simulink model "WEC_Sim_Driver"  (R2013a)
settings: Solver=ode4  StartTime=StartTime  StopTime=EndTime  FixedStep=deltaT  MaxStep=deltaTMax  MinStep=deltaTMin  RelTol=1e-3
undefined symbols (not defined in the file): A_bore, A_c_F, A_c_P, A_rod, angle_arm_aft, Bd, C_aft, deltaT, Gen_Damp, hyd_mot_eff, hydro, hydroForce, Jtot, K_aft, Kd, mooring_c, mooring_k, nonlinear_params, omega_s, p_atm, p_hp, p_lp, pump_vol_eff, r_g, STLfloat, STLplate, Ts, V_hp, V_lp, Vg, X, Y, Z
libraries: nesl_utility x35, sm_lib x14
(part 2 of 2)

== matlab function WEC_Sim_Driver/Structure2/Convert ==
  data: Q input; E output
function E  = EulerAngle(Q)
%#codegen
E=zeros(3,1);
E(1) = atan( (2*(Q(1)*Q(2)+Q(3)*Q(4))) / (1-2* (Q(2)^2+Q(3)^2) ) );
E(2) = asin( 2* (Q(1)*Q(3) - Q(4)*Q(2)));
E(3) = atan( (2*(Q(1)*Q(4)+Q(2)*Q(3))) / (1-2* (Q(3)^2+Q(4)^2) ) );

== matlab function WEC_Sim_Driver/Structure2/Convert1 ==
  data: Q input; E output
function E  = EulerAngle(Q)
%#codegen
E=zeros(3,1);
E(1) = atan( (2*(Q(1)*Q(2)+Q(3)*Q(4))) / (1-2* (Q(2)^2+Q(3)^2) ) );
E(2) = asin( 2* (Q(1)*Q(3) - Q(4)*Q(2)));
E(3) = atan( (2*(Q(1)*Q(4)+Q(2)*Q(3))) / (1-2* (Q(3)^2+Q(4)^2) ) );

== matlab function WEC_Sim_Driver/Structure2/Convert2 ==
  data: Q input; E output
function E  = EulerAngle(Q)
%#codegen
E=zeros(3,1);
E(1) = atan( (2*(Q(1)*Q(2)+Q(3)*Q(4))) / (1-2* (Q(2)^2+Q(3)^2) ) );
E(2) = asin( 2* (Q(1)*Q(3) - Q(4)*Q(2)));
E(3) = atan( (2*(Q(1)*Q(4)+Q(2)*Q(3))) / (1-2* (Q(3)^2+Q(4)^2) ) );

== matlab function WEC_Sim_Driver/Linear HydroForce2/MATLAB Function ==
  data: t input; F output; deltaT input; matrix input
function F  = ExcitationLookup(t,deltaT,matrix)

int=round(t/deltaT+1);
F=matrix(int,:)';

== matlab function WEC_Sim_Driver/Fully-Nonlinear HydroForce2/Linear Excitation ==
  data: t input; F output; deltaT input; matrix input
function F  = ExcitationLookup(t,deltaT,matrix)

int=round(t/deltaT+1);
F=matrix(int,:)';

== matlab function WEC_Sim_Driver/Fully-Nonlinear HydroForce1/Fully-Nonlinear Hydrostatic Restoring and Excitation/Body1 Nonlinear Restoring and Excitation ==
  data: STL input; t input; BodyForce output; Disp input; BodyMoment output; nonlinear_params input; psi_m output; p_FK_total output; p_FK_l_total output
function [BodyForce,BodyMoment,psi_m,p_FK_total,p_FK_l_total] = vectorbuoyancy(STL, t,Disp,nonlinear_params)
%STL(a,b,c)  where a denotes the triangle, b denotes the point (1-3) and c
%            denotes the component (x, y or z)
%dZ          a scalar value describing HEAVE
%axisRot     a vector describing the axis about which the body is rotated
%angleRot    the angle by which the body is rotated about axisRot
%refZ        the location of the

% algorithm for point rotation from http://paulbourke.net/geometry/rotate/
% algorithm for volume calc from
% http://stackoverflow.com/questions/1406029/how-to-calculate-the-volume-of-a-3d-mesh-object-the-surface-of-which-is-made-up
% via  http://amp.ece.cmu.edu/Publication/Cha/icip01_Cha.pdf

%determine size of STL
[a b c] = size(STL);

%make sure angleRot is a unit vector
% magAR = sqrt(axisRot(1)^2 + axisRot(2)^2 + axisRot(3)^2);
% axisRot = axisRot/magAR;
axisRotx=[1 0 0];
axisRoty=[0 1 0];
dX=Disp(1);
dZ=Disp(3);
angleRotx=Disp(4);
angleRoty=Disp(5);
Amp=nonlinear_params(1);
k=nonlinear_params(2);
w=nonlinear_params(3);
d=nonlinear_params(4);
psi = zeros(a,b);
psi_l= zeros(a,b);
psi_m = 0;
psi_avg = zeros(a,b);
psi_l_avg = zeros(a,b);
STL_l=zeros(size(STL));

% Fix body at mean water level for linear buoyancy & excitation calc
for i=1:1:a
    for j=1:1:3
        q_l = zeros(1,3);
            %plunge object
            q_l(1) = STL(i,j,1);
            q_l(2) = STL(i,j,2);
            q_l(3) = STL(i,j,3) -17.606;
        if q_l(3) > 0
            q_l(3) = 0;
        end
        psi_l(i,j) =Amp*cos(k*(q_l(1)+dX)-w*t);
        %save altered point
        STL_l(i,j,:) = q_l;
    end
end

% Rotate and translate body for nonlinear buoyancy & excitation calc
for i=1:1:a
    for j=1:1:3
        q = zeros(1,3);
        
        %Calculate water height near body CG before moving body
        if STL(i,j,1)<0.001
            psi_m=Amp*cos(k*(dX)-w*t);
        end
        
%         perform y-direction rotation
        if angleRoty ~= 0
            
            costhetay = cos(angleRoty);
            sinthetay = sin(angleRoty);
            
            q(1) = q(1) + (costhetay + (1 - costhetay) * axisRoty(1) * axisRoty(1)) * STL(i,j,1);
            q(1) = q(1) + ((1 - costhetay) * axisRoty(1) * axisRoty(2) - axisRoty(3) * sinthetay) * STL(i,j,2);
            q(1) = q(1) + ((1 - costhetay) * axisRoty(1) * axisRoty(3) + axisRoty(2) * sinthetay) * STL(i,j,3);
            
            q(2) = q(2) + ((1 - costhetay) * axisRoty(1) * axisRoty(2) + axisRoty(3) * sinthetay) * STL(i,j,1);
            q(2) = q(2) + (costhetay + (1 - costhetay) * axisRoty(2) * axisRoty(2)) * STL(i,j,2);
            q(2) = q(2) + ((1 - costhetay) * axisRoty(2) * axisRoty(3) - axisRoty(1) * sinthetay) * STL(i,j,3);
            
            q(3) = q(3) + ((1 - costhetay) * axisRoty(1) * axisRoty(3) - axisRoty(2) * sinthetay) * STL(i,j,1);
            q(3) = q(3) + ((1 - costhetay) * axisRoty(2) * axisRoty(3) + axisRoty(1) * sinthetay) * STL(i,j,2);
            q(3) = q(3) + (costhetay + (1 - costhetay) * axisRoty(3) * axisRoty(3)) * STL(i,j,3);
            
%             q(3) = q(3) + dZ(1);
        end
        if angleRoty ~= 0
        %save altered point
        STL(i,j,:) = q;
        end
    end
end

for i=1:1:a
    for j=1:1:3
        q = zeros(1,3);
%         %perform x-direction rotation
        if angleRotx ~= 0
            
            costhetax = cos(angleRotx);
            sinthetax = sin(angleRotx);
            
            q(1) = q(1) + (costhetax + (1 - costhetax) * axisRotx(1) * axisRotx(1)) * STL(i,j,1);
            q(1) = q(1) + ((1 - costhetax) * axisRotx(1) * axisRotx(2) - axisRotx(3) * sinthetax) * STL(i,j,2);
            q(1) = q(1) + ((1 - costhetax) * axisRotx(1) * axisRotx(3) + axisRotx(2) * sinthetax) * STL(i,j,3);
            
            q(2) = q(2) + ((1 - costhetax) * axisRotx(1) * axisRotx(2) + axisRotx(3) * sinthetax) * STL(i,j,1);
            q(2) = q(2) + (costhetax + (1 - costhetax) * axisRotx(2) * axisRotx(2)) * STL(i,j,2);
            q(2) = q(2) + ((1 - costhetax) * axisRotx(2) * axisRotx(3) - axisRotx(1) * sinthetax) * STL(i,j,3);
            
            q(3) = q(3) + ((1 - costhetax) * axisRotx(1) * axisRotx(3) - axisRotx(2) * sinthetax) * STL(i,j,1);
            q(3) = q(3) + ((1 - costhetax) * axisRotx(2) * axisRotx(3) + axisRotx(1) * sinthetax) * STL(i,j,2);
            q(3) = q(3) + (costhetax + (1 - costhetax) * axisRotx(3) * axisRotx(3)) * STL(i,j,3);
            
            q(3) = q(3) + dZ(1);
        else
            %plunge object
            q(1) = STL(i,j,1);
            q(2) = STL(i,j,2);
            q(3) = STL(i,j,3) + dZ(1);
        end
        
        %Truncate at instantaneous free surface
        psi(i,j) =Amp*cos(k*(q(1)+ dX)-w*t);
        if q(3) > psi(i,j)
            q(3) = psi(i,j);
        end
        
        %Truncate at instantaneous free surface
%         if q(3) > 0
%             q(3) = 0;
%         end
        
        %save altered point
        STL(i,j,:) = q;
    end
end

%Calculate buoyancy force and restoring moments
BodyForce=zeros(3,1);
BodyMoment=zeros(3,1);
p_FK_total=zeros(3,1);
p_FK_l_total=zeros(3,1);
for i=1:1:a
    x_m=(STL(i,1,1)+STL(i,2,1)+STL(i,3,1))/3;        %z coordinate for panel center
    y_m=(STL(i,1,2)+STL(i,2,2)+STL(i,3,2))/3;        %z coordinate for panel center
    z_m=(STL(i,1,3)+STL(i,2,3)+STL(i,3,3))/3;        %z coordinate for panel center
    r_m=[x_m; y_m; z_m];
        
    r_a=[STL(i,1,1); STL(i,1,2); STL(i,1,3)];             %vector describing location of panel's A vertex
    r_b=[STL(i,2,1); STL(i,2,2); STL(i,2,3)];             %vector describing location of panel's B vertex
    r_c=[STL(i,3,1); STL(i,3,2); STL(i,3,3)];             %vector describing location of panel's C vertex
 
    AB=r_b-r_a;
    AC=r_c-r_a;
    CP=cross(AC,AB);
    area=.5*CP;
    
    x_m_l=(STL_l(i,1,1)+STL_l(i,2,1)+STL_l(i,3,1))/3;        %z coordinate for panel center
    y_m_l=(STL_l(i,1,2)+STL_l(i,2,2)+STL_l(i,3,2))/3;        %z coordinate for panel center
    z_m_l=(STL_l(i,1,3)+STL_l(i,2,3)+STL_l(i,3,3))/3;        %z coordinate for panel center
    r_m_l=[x_m_l; y_m_l; z_m_l];  
    
    r_a_l=[STL_l(i,1,1); STL_l(i,1,2); STL_l(i,1,3)];             %vector describing location of panel's A vertex
    r_b_l=[STL_l(i,2,1); STL_l(i,2,2); STL_l(i,2,3)];             %vector describing location of panel's B vertex
    r_c_l=[STL_l(i,3,1); STL_l(i,3,2); STL_l(i,3,3)];             %vector describing location of panel's C verte
      
    AB_l=r_b_l-r_a_l;
    AC_l=r_c_l-r_a_l;
    CP_l=cross(AC_l,AB_l);
    area_l=.5*CP_l;
    
    psi_avg = (psi(i,1)+psi(i,2)+psi(i,3))/3;
    psi_l_avg = (psi_l(i,1)+psi_l(i,2)+psi_l(i,3))/3;
    
    p_HS=-z_m*area;
    p_FK=area*psi_avg*cosh(k*(z_m+psi_avg+d))/cosh(k*d);
    p_FK_l=area_l*psi_l_avg*cosh(k*(z_m_l+psi_l_avg+d))/cosh(k*d);
    p_total=p_HS+p_FK-p_FK_l;
    
    BodyForce=BodyForce+p_total;
    PanelMoment=cross(r_m,p_total);
    BodyMoment=BodyMoment+PanelMoment;

    p_FK_total=p_FK_total+p_FK;
    p_FK_l_total=p_FK_l_total+p_FK_l;
end
% BodyForce(1)=0;
% BodyForce(2)=0;
% BodyMoment(1)=-0.05*angleRot(1);
% BodyMoment(3)=-50000*angleRot(3);

== matlab function WEC_Sim_Driver/Fully-Nonlinear HydroForce1/Linear Excitation ==
  data: t input; F output; deltaT input; matrix input
function F  = ExcitationLookup(t,deltaT,matrix)

int=round(t/deltaT+1);
F=matrix(int,:)';

== matlab function WEC_Sim_Driver/Quasi-Nonlinear HydroForce2/Linear Excitation ==
  data: t input; F output; deltaT input; matrix input
function F  = ExcitationLookup(t,deltaT,matrix)

int=round(t/deltaT+1);
F=matrix(int,:)';

== matlab function WEC_Sim_Driver/Quasi-Nonlinear HydroForce2/Quasi-Nonlinear Hydrostatic Restoring/Submerged Volume ==
  data: STL input; BodyForce output; Disp2 input; BodyMoment output; TotalArea output; PanelForce output
function [BodyForce,BodyMoment,TotalArea,PanelForce] = vectorbuoyancy(STL, Disp2)
%STL(a,b,c)  where a denotes the triangle, b denotes the point (1-3) and c
%            denotes the component (x, y or z)
%dZ          a scalar value describing HEAVE
%axisRot     a vector describing the axis about which the body is rotated
%angleRot    the angle by which the body is rotated about axisRot
%refZ        the location of the

% algorithm for point rotation from http://paulbourke.net/geometry/rotate/
% algorithm for volume calc from
% http://stackoverflow.com/questions/1406029/how-to-calculate-the-volume-of-a-3d-mesh-object-the-surface-of-which-is-made-up
% via  http://amp.ece.cmu.edu/Publication/Cha/icip01_Cha.pdf

%determine size of STL
[a b c] = size(STL);

%make sure angleRot is a unit vector
% magAR = sqrt(axisRot(1)^2 + axisRot(2)^2 + axisRot(3)^2);
% axisRot = axisRot/magAR;
axisRotx=[1 0 0];
axisRoty=[0 1 0];
dZ=Disp2(3);
angleRotx=Disp2(4);
angleRoty=Disp2(5);

% update locations of points
for i=1:1:a
    for j=1:1:3
        q = zeros(1,3);
        
%         perform y-direction rotation
        if angleRoty ~= 0
            
            costhetay = cos(angleRoty);
            sinthetay = sin(angleRoty);
            
            q(1) = q(1) + (costhetay + (1 - costhetay) * axisRoty(1) * axisRoty(1)) * STL(i,j,1);
            q(1) = q(1) + ((1 - costhetay) * axisRoty(1) * axisRoty(2) - axisRoty(3) * sinthetay) * STL(i,j,2);
            q(1) = q(1) + ((1 - costhetay) * axisRoty(1) * axisRoty(3) + axisRoty(2) * sinthetay) * STL(i,j,3);
            
            q(2) = q(2) + ((1 - costhetay) * axisRoty(1) * axisRoty(2) + axisRoty(3) * sinthetay) * STL(i,j,1);
            q(2) = q(2) + (costhetay + (1 - costhetay) * axisRoty(2) * axisRoty(2)) * STL(i,j,2);
            q(2) = q(2) + ((1 - costhetay) * axisRoty(2) * axisRoty(3) - axisRoty(1) * sinthetay) * STL(i,j,3);
            
            q(3) = q(3) + ((1 - costhetay) * axisRoty(1) * axisRoty(3) - axisRoty(2) * sinthetay) * STL(i,j,1);
            q(3) = q(3) + ((1 - costhetay) * axisRoty(2) * axisRoty(3) + axisRoty(1) * sinthetay) * STL(i,j,2);
            q(3) = q(3) + (costhetay + (1 - costhetay) * axisRoty(3) * axisRoty(3)) * STL(i,j,3);
            
%             q(3) = q(3) + dZ(1);
        end
        if angleRoty ~= 0
        %save altered point
        STL(i,j,:) = q;
        end
    end
end

for i=1:1:a
    for j=1:1:3
        q = zeros(1,3);
%         %perform x-direction rotation
        if angleRotx ~= 0
            
            costhetax = cos(angleRotx);
            sinthetax = sin(angleRotx);
            
            q(1) = q(1) + (costhetax + (1 - costhetax) * axisRotx(1) * axisRotx(1)) * STL(i,j,1);
            q(1) = q(1) + ((1 - costhetax) * axisRotx(1) * axisRotx(2) - axisRotx(3) * sinthetax) * STL(i,j,2);
            q(1) = q(1) + ((1 - costhetax) * axisRotx(1) * axisRotx(3) + axisRotx(2) * sinthetax) * STL(i,j,3);
            
            q(2) = q(2) + ((1 - costhetax) * axisRotx(1) * axisRotx(2) + axisRotx(3) * sinthetax) * STL(i,j,1);
            q(2) = q(2) + (costhetax + (1 - costhetax) * axisRotx(2) * axisRotx(2)) * STL(i,j,2);
            q(2) = q(2) + ((1 - costhetax) * axisRotx(2) * axisRotx(3) - axisRotx(1) * sinthetax) * STL(i,j,3);
            
            q(3) = q(3) + ((1 - costhetax) * axisRotx(1) * axisRotx(3) - axisRotx(2) * sinthetax) * STL(i,j,1);
            q(3) = q(3) + ((1 - costhetax) * axisRotx(2) * axisRotx(3) + axisRotx(1) * sinthetax) * STL(i,j,2);
            q(3) = q(3) + (costhetax + (1 - costhetax) * axisRotx(3) * axisRotx(3)) * STL(i,j,3);
            
            q(3) = q(3) + dZ(1);
        else
            %plunge object
            q(1) = STL(i,j,1);
            q(2) = STL(i,j,2);
            q(3) = STL(i,j,3) + dZ(1);
        end
        
        %truncate at water surface
        if q(3) > 0
            q(3) = 0;
        end
        
        %save altered point
        STL(i,j,:) = q;
    end
end

%Calculate buoyancy force and restoring moments
BodyForce=zeros(3,1);
BodyMoment=zeros(3,1);
TotalArea=zeros(3,1);
for i=1:1:a
    x_m=(STL(i,1,1)+STL(i,2,1)+STL(i,3,1))/3;        %z coordinate for panel center
    y_m=(STL(i,1,2)+STL(i,2,2)+STL(i,3,2))/3;        %z coordinate for panel center
    z_m=(STL(i,1,3)+STL(i,2,3)+STL(i,3,3))/3;        %z coordinate for panel center
    r_m=[x_m; y_m; z_m];
        
    r_a=[STL(i,1,1); STL(i,1,2); STL(i,1,3)];             %vector describing location of panel's A vertex
    r_b=[STL(i,2,1); STL(i,2,2); STL(i,2,3)];             %vector describing location of panel's B vertex
    r_c=[STL(i,3,1); STL(i,3,2); STL(i,3,3)];             %vector describing location of panel's C vertex
 
    AB=r_b-r_a;
    AC=r_c-r_a;
    CP=cross(AC,AB);
    area=.5*CP;
    
    PanelForce=-z_m*area;
    BodyForce=BodyForce+PanelForce;
    
    PanelMoment=cross(r_m,PanelForce);
    BodyMoment=BodyMoment+PanelMoment;
    TotalArea=TotalArea+area;
end

% BodyForce(1)=0;
% BodyForce(2)=0;
% BodyMoment(1)=-0.05*angleRot(1);
% BodyMoment(3)=-50000*angleRot(3);

== matlab function WEC_Sim_Driver/Fully-Nonlinear HydroForce2/Fully-Nonlinear Hydrostatic Restoring and Excitation/Body1 Nonlinear Restoring and Excitation ==
  data: STL input; t input; BodyForce output; Disp2 input; BodyMoment output; nonlinear_params input; psi_m output; p_FK_total output; p_FK_l_total output
function [BodyForce,BodyMoment,psi_m,p_FK_total,p_FK_l_total] = vectorbuoyancy(STL, t,Disp2,nonlinear_params)
%STL(a,b,c)  where a denotes the triangle, b denotes the point (1-3) and c
%            denotes the component (x, y or z)
%dZ          a scalar value describing HEAVE
%axisRot     a vector describing the axis about which the body is rotated
%angleRot    the angle by which the body is rotated about axisRot
%refZ        the location of the

% algorithm for point rotation from http://paulbourke.net/geometry/rotate/
% algorithm for volume calc from
% http://stackoverflow.com/questions/1406029/how-to-calculate-the-volume-of-a-3d-mesh-object-the-surface-of-which-is-made-up
% via  http://amp.ece.cmu.edu/Publication/Cha/icip01_Cha.pdf

%determine size of STL
[a b c] = size(STL);

%make sure angleRot is a unit vector
% magAR = sqrt(axisRot(1)^2 + axisRot(2)^2 + axisRot(3)^2);
% axisRot = axisRot/magAR;
axisRotx=[1 0 0];
axisRoty=[0 1 0];
dX=Disp2(1);
dZ=Disp2(3);
angleRotx=Disp2(4);
angleRoty=Disp2(5);
Amp=nonlinear_params(1);
k=nonlinear_params(2);
w=nonlinear_params(3);
d=nonlinear_params(4);
psi = zeros(a,b);
psi_l= zeros(a,b);
psi_m = 0;
psi_avg = zeros(a,b);
psi_l_avg = zeros(a,b);
STL_l=zeros(size(STL));

% Fix body at mean water level for linear buoyancy & excitation calc
for i=1:1:a
    for j=1:1:3
        q_l = zeros(1,3);
            %plunge object
            q_l(1) = STL(i,j,1);
            q_l(2) = STL(i,j,2);
            q_l(3) = STL(i,j,3) -17.606;
        if q_l(3) > 0
            q_l(3) = 0;
        end
        psi_l(i,j) =Amp*cos(k*(q_l(1)+dX)-w*t);
        %save altered point
        STL_l(i,j,:) = q_l;
    end
end

% Rotate and translate body for nonlinear buoyancy & excitation calc
for i=1:1:a
    for j=1:1:3
        q = zeros(1,3);
        
        %Calculate water height near body CG before moving body
        if STL(i,j,1)<0.001
            psi_m=Amp*cos(k*(dX)-w*t);
        end
        
%         perform y-direction rotation
        if angleRoty ~= 0
            
            costhetay = cos(angleRoty);
            sinthetay = sin(angleRoty);
            
            q(1) = q(1) + (costhetay + (1 - costhetay) * axisRoty(1) * axisRoty(1)) * STL(i,j,1);
            q(1) = q(1) + ((1 - costhetay) * axisRoty(1) * axisRoty(2) - axisRoty(3) * sinthetay) * STL(i,j,2);
            q(1) = q(1) + ((1 - costhetay) * axisRoty(1) * axisRoty(3) + axisRoty(2) * sinthetay) * STL(i,j,3);
            
            q(2) = q(2) + ((1 - costhetay) * axisRoty(1) * axisRoty(2) + axisRoty(3) * sinthetay) * STL(i,j,1);
            q(2) = q(2) + (costhetay + (1 - costhetay) * axisRoty(2) * axisRoty(2)) * STL(i,j,2);
            q(2) = q(2) + ((1 - costhetay) * axisRoty(2) * axisRoty(3) - axisRoty(1) * sinthetay) * STL(i,j,3);
            
            q(3) = q(3) + ((1 - costhetay) * axisRoty(1) * axisRoty(3) - axisRoty(2) * sinthetay) * STL(i,j,1);
            q(3) = q(3) + ((1 - costhetay) * axisRoty(2) * axisRoty(3) + axisRoty(1) * sinthetay) * STL(i,j,2);
            q(3) = q(3) + (costhetay + (1 - costhetay) * axisRoty(3) * axisRoty(3)) * STL(i,j,3);
            
%             q(3) = q(3) + dZ(1);
        end
        if angleRoty ~= 0
        %save altered point
        STL(i,j,:) = q;
        end
    end
end

for i=1:1:a
    for j=1:1:3
        q = zeros(1,3);
%         %perform x-direction rotation
        if angleRotx ~= 0
            
            costhetax = cos(angleRotx);
            sinthetax = sin(angleRotx);
            
            q(1) = q(1) + (costhetax + (1 - costhetax) * axisRotx(1) * axisRotx(1)) * STL(i,j,1);
            q(1) = q(1) + ((1 - costhetax) * axisRotx(1) * axisRotx(2) - axisRotx(3) * sinthetax) * STL(i,j,2);
            q(1) = q(1) + ((1 - costhetax) * axisRotx(1) * axisRotx(3) + axisRotx(2) * sinthetax) * STL(i,j,3);
            
            q(2) = q(2) + ((1 - costhetax) * axisRotx(1) * axisRotx(2) + axisRotx(3) * sinthetax) * STL(i,j,1);
            q(2) = q(2) + (costhetax + (1 - costhetax) * axisRotx(2) * axisRotx(2)) * STL(i,j,2);
            q(2) = q(2) + ((1 - costhetax) * axisRotx(2) * axisRotx(3) - axisRotx(1) * sinthetax) * STL(i,j,3);
            
            q(3) = q(3) + ((1 - costhetax) * axisRotx(1) * axisRotx(3) - axisRotx(2) * sinthetax) * STL(i,j,1);
            q(3) = q(3) + ((1 - costhetax) * axisRotx(2) * axisRotx(3) + axisRotx(1) * sinthetax) * STL(i,j,2);
            q(3) = q(3) + (costhetax + (1 - costhetax) * axisRotx(3) * axisRotx(3)) * STL(i,j,3);
            
            q(3) = q(3) + dZ(1);
        else
            %plunge object
            q(1) = STL(i,j,1);
            q(2) = STL(i,j,2);
            q(3) = STL(i,j,3) + dZ(1);
        end
        
        %Truncate at instantaneous free surface
        psi(i,j) =Amp*cos(k*(q(1)+ dX)-w*t);
        if q(3) > psi(i,j)
            q(3) = psi(i,j);
        end
        
        %Truncate at instantaneous free surface
%         if q(3) > 0
%             q(3) = 0;
%         end
        
        %save altered point
        STL(i,j,:) = q;
    end
end

%Calculate buoyancy force and restoring moments
BodyForce=zeros(3,1);
BodyMoment=zeros(3,1);
p_FK_total=zeros(3,1);
p_FK_l_total=zeros(3,1);
for i=1:1:a
    x_m=(STL(i,1,1)+STL(i,2,1)+STL(i,3,1))/3;        %z coordinate for panel center
    y_m=(STL(i,1,2)+STL(i,2,2)+STL(i,3,2))/3;        %z coordinate for panel center
    z_m=(STL(i,1,3)+STL(i,2,3)+STL(i,3,3))/3;        %z coordinate for panel center
    r_m=[x_m; y_m; z_m];
        
    r_a=[STL(i,1,1); STL(i,1,2); STL(i,1,3)];             %vector describing location of panel's A vertex
    r_b=[STL(i,2,1); STL(i,2,2); STL(i,2,3)];             %vector describing location of panel's B vertex
    r_c=[STL(i,3,1); STL(i,3,2); STL(i,3,3)];             %vector describing location of panel's C vertex
 
    AB=r_b-r_a;
    AC=r_c-r_a;
    CP=cross(AC,AB);
    area=.5*CP;
    
    x_m_l=(STL_l(i,1,1)+STL_l(i,2,1)+STL_l(i,3,1))/3;        %z coordinate for panel center
    y_m_l=(STL_l(i,1,2)+STL_l(i,2,2)+STL_l(i,3,2))/3;        %z coordinate for panel center
    z_m_l=(STL_l(i,1,3)+STL_l(i,2,3)+STL_l(i,3,3))/3;        %z coordinate for panel center
    r_m_l=[x_m_l; y_m_l; z_m_l];  
    
    r_a_l=[STL_l(i,1,1); STL_l(i,1,2); STL_l(i,1,3)];             %vector describing location of panel's A vertex
    r_b_l=[STL_l(i,2,1); STL_l(i,2,2); STL_l(i,2,3)];             %vector describing location of panel's B vertex
    r_c_l=[STL_l(i,3,1); STL_l(i,3,2); STL_l(i,3,3)];             %vector describing location of panel's C verte
      
    AB_l=r_b_l-r_a_l;
    AC_l=r_c_l-r_a_l;
    CP_l=cross(AC_l,AB_l);
    area_l=.5*CP_l;
    
    psi_avg = (psi(i,1)+psi(i,2)+psi(i,3))/3;
    psi_l_avg = (psi_l(i,1)+psi_l(i,2)+psi_l(i,3))/3;
    
    p_HS=-z_m*area;
    p_FK=area*psi_avg*cosh(k*(z_m+psi_avg+d))/cosh(k*d);
    p_FK_l=area_l*psi_l_avg*cosh(k*(z_m_l+psi_l_avg+d))/cosh(k*d);
    p_total=p_HS+p_FK-p_FK_l;
    
    BodyForce=BodyForce+p_total;
    PanelMoment=cross(r_m,p_total);
    BodyMoment=BodyMoment+PanelMoment;

    p_FK_total=p_FK_total+p_FK;
    p_FK_l_total=p_FK_l_total+p_FK_l;
end
% BodyForce(1)=0;
% BodyForce(2)=0;
% BodyMoment(1)=-0.05*angleRot(1);
% BodyMoment(3)=-50000*angleRot(3);

== matlab function WEC_Sim_Driver/Linear HydroForce1/MATLAB Function ==
  data: t input; F output; deltaT input; matrix input
function F  = ExcitationLookup(t,deltaT,matrix)

int=round(t/deltaT+1);
F=matrix(int,:)';

== matlab function WEC_Sim_Driver/Structure1/Convert ==
  data: Q input; E output
function E  = EulerAngle(Q)
%#codegen
E=zeros(3,1);
E(1) = atan( (2*(Q(1)*Q(2)+Q(3)*Q(4))) / (1-2* (Q(2)^2+Q(3)^2) ) );
E(2) = asin( 2* (Q(1)*Q(3) - Q(4)*Q(2)));
E(3) = atan( (2*(Q(1)*Q(4)+Q(2)*Q(3))) / (1-2* (Q(3)^2+Q(4)^2) ) );

== matlab function WEC_Sim_Driver/Quasi-Nonlinear HydroForce1/Linear Excitation ==
  data: t input; F output; deltaT input; matrix input
function F  = ExcitationLookup(t,deltaT,matrix)

int=round(t/deltaT+1);
F=matrix(int,:)';

== matlab function WEC_Sim_Driver/Quasi-Nonlinear HydroForce1/Quasi-Nonlinear Hydrostatic Restoring/Submerged Volume ==
  data: STL input; BodyForce output; Disp input; BodyMoment output; TotalArea output; PanelForce output
function [BodyForce,BodyMoment,TotalArea,PanelForce] = vectorbuoyancy(STL, Disp)
%STL(a,b,c)  where a denotes the triangle, b denotes the point (1-3) and c
%            denotes the component (x, y or z)
%dZ          a scalar value describing HEAVE
%axisRot     a vector describing the axis about which the body is rotated
%angleRot    the angle by which the body is rotated about axisRot
%refZ        the location of the

% algorithm for point rotation from http://paulbourke.net/geometry/rotate/
% algorithm for volume calc from
% http://stackoverflow.com/questions/1406029/how-to-calculate-the-volume-of-a-3d-mesh-object-the-surface-of-which-is-made-up
% via  http://amp.ece.cmu.edu/Publication/Cha/icip01_Cha.pdf

%determine size of STL
[a b c] = size(STL);

%make sure angleRot is a unit vector
% magAR = sqrt(axisRot(1)^2 + axisRot(2)^2 + axisRot(3)^2);
% axisRot = axisRot/magAR;
axisRotx=[1 0 0];
axisRoty=[0 1 0];
dZ=Disp(3);
angleRotx=Disp(4);
angleRoty=Disp(5);

% update locations of points
for i=1:1:a
    for j=1:1:3
        q = zeros(1,3);
        
%         perform y-direction rotation
        if angleRoty ~= 0
            
            costhetay = cos(angleRoty);
            sinthetay = sin(angleRoty);
            
            q(1) = q(1) + (costhetay + (1 - costhetay) * axisRoty(1) * axisRoty(1)) * STL(i,j,1);
            q(1) = q(1) + ((1 - costhetay) * axisRoty(1) * axisRoty(2) - axisRoty(3) * sinthetay) * STL(i,j,2);
            q(1) = q(1) + ((1 - costhetay) * axisRoty(1) * axisRoty(3) + axisRoty(2) * sinthetay) * STL(i,j,3);
            
            q(2) = q(2) + ((1 - costhetay) * axisRoty(1) * axisRoty(2) + axisRoty(3) * sinthetay) * STL(i,j,1);
            q(2) = q(2) + (costhetay + (1 - costhetay) * axisRoty(2) * axisRoty(2)) * STL(i,j,2);
            q(2) = q(2) + ((1 - costhetay) * axisRoty(2) * axisRoty(3) - axisRoty(1) * sinthetay) * STL(i,j,3);
            
            q(3) = q(3) + ((1 - costhetay) * axisRoty(1) * axisRoty(3) - axisRoty(2) * sinthetay) * STL(i,j,1);
            q(3) = q(3) + ((1 - costhetay) * axisRoty(2) * axisRoty(3) + axisRoty(1) * sinthetay) * STL(i,j,2);
            q(3) = q(3) + (costhetay + (1 - costhetay) * axisRoty(3) * axisRoty(3)) * STL(i,j,3);
            
%             q(3) = q(3) + dZ(1);
        end
        if angleRoty ~= 0
        %save altered point
        STL(i,j,:) = q;
        end
    end
end

for i=1:1:a
    for j=1:1:3
        q = zeros(1,3);
%         %perform x-direction rotation
        if angleRotx ~= 0
            
            costhetax = cos(angleRotx);
            sinthetax = sin(angleRotx);
            
            q(1) = q(1) + (costhetax + (1 - costhetax) * axisRotx(1) * axisRotx(1)) * STL(i,j,1);
            q(1) = q(1) + ((1 - costhetax) * axisRotx(1) * axisRotx(2) - axisRotx(3) * sinthetax) * STL(i,j,2);
            q(1) = q(1) + ((1 - costhetax) * axisRotx(1) * axisRotx(3) + axisRotx(2) * sinthetax) * STL(i,j,3);
            
            q(2) = q(2) + ((1 - costhetax) * axisRotx(1) * axisRotx(2) + axisRotx(3) * sinthetax) * STL(i,j,1);
            q(2) = q(2) + (costhetax + (1 - costhetax) * axisRotx(2) * axisRotx(2)) * STL(i,j,2);
            q(2) = q(2) + ((1 - costhetax) * axisRotx(2) * axisRotx(3) - axisRotx(1) * sinthetax) * STL(i,j,3);
            
            q(3) = q(3) + ((1 - costhetax) * axisRotx(1) * axisRotx(3) - axisRotx(2) * sinthetax) * STL(i,j,1);
            q(3) = q(3) + ((1 - costhetax) * axisRotx(2) * axisRotx(3) + axisRotx(1) * sinthetax) * STL(i,j,2);
            q(3) = q(3) + (costhetax + (1 - costhetax) * axisRotx(3) * axisRotx(3)) * STL(i,j,3);
            
            q(3) = q(3) + dZ(1);
        else
            %plunge object
            q(1) = STL(i,j,1);
            q(2) = STL(i,j,2);
            q(3) = STL(i,j,3) + dZ(1);
        end
        
        %truncate at water surface
        if q(3) > 0
            q(3) = 0;
        end
        
        %save altered point
        STL(i,j,:) = q;
    end
end

%Calculate buoyancy force and restoring moments
BodyForce=zeros(3,1);
BodyMoment=zeros(3,1);
TotalArea=zeros(3,1);
for i=1:1:a
    x_m=(STL(i,1,1)+STL(i,2,1)+STL(i,3,1))/3;        %z coordinate for panel center
    y_m=(STL(i,1,2)+STL(i,2,2)+STL(i,3,2))/3;        %z coordinate for panel center
    z_m=(STL(i,1,3)+STL(i,2,3)+STL(i,3,3))/3;        %z coordinate for panel center
    r_m=[x_m; y_m; z_m];
        
    r_a=[STL(i,1,1); STL(i,1,2); STL(i,1,3)];             %vector describing location of panel's A vertex
    r_b=[STL(i,2,1); STL(i,2,2); STL(i,2,3)];             %vector describing location of panel's B vertex
    r_c=[STL(i,3,1); STL(i,3,2); STL(i,3,3)];             %vector describing location of panel's C vertex
 
    AB=r_b-r_a;
    AC=r_c-r_a;
    CP=cross(AC,AB);
    area=.5*CP;
    
    PanelForce=-z_m*area;
    BodyForce=BodyForce+PanelForce;
    
    PanelMoment=cross(r_m,PanelForce);
    BodyMoment=BodyMoment+PanelMoment;
    TotalArea=TotalArea+area;
end

% BodyForce(1)=0;
% BodyForce(2)=0;
% BodyMoment(1)=-0.05*angleRot(1);
% BodyMoment(3)=-50000*angleRot(3);
